simulink model "dual_mass_plant"  (R2023a)
settings: Solver=VariableStepAuto  StartTime=0.0  StopTime=50  RelTol=1e-3
values from neighbouring files (symbols this model uses):
  C = [1 0 1 0]    [dual_param.m]
  Kf1 = 2.0    (= 2)    [dual_param.m]
  Kf2 = 10.0    (= 10)    [dual_param.m]
  Kv1 = 0.1    [dual_param.m]
  Kv2 = 0.5    [dual_param.m]
  M = 10.0    (= 10)    [dual_param.m]
  m = 1.0    (= 1)    [dual_param.m]
  U1 = 1.0    (= 1)    [dual_param.m]
  U2 = 3.0    (= 3)    [dual_param.m]
settings Model: Creator=Admin  LastModifiedBy=Admin
settings ModelReferenceCC: EnableRefExpFcnMdlSchedulingChecks=on

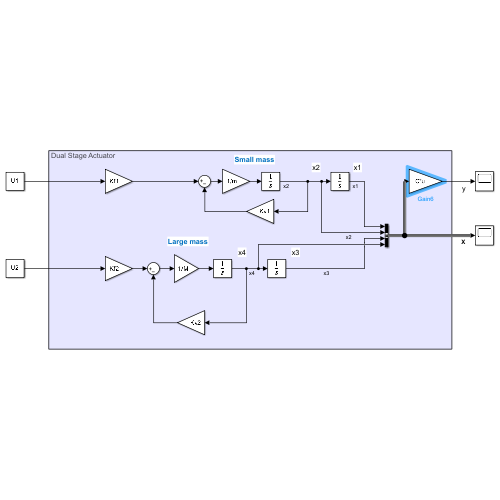
[thumbnail: Simulink's stored preview of the top-level diagram]
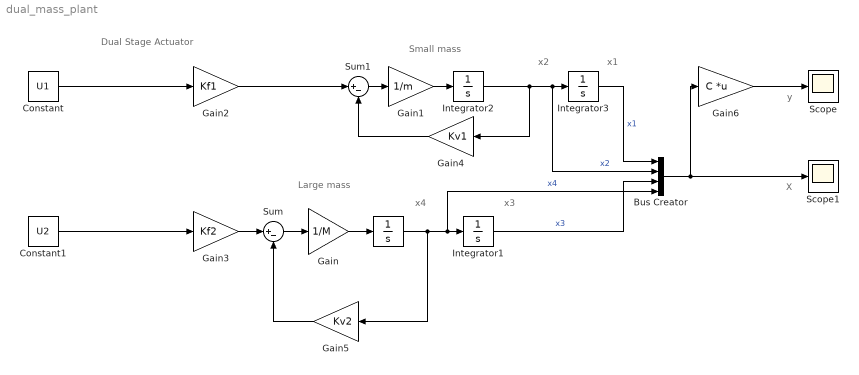
== system dual_mass_plant ==
  note: X
  note: Dual Stage Actuator
  note: y
  note: Small mass
  note: Large mass
  note: x1
  note: x2
  note: x3
  note: x4
  " " : Integrator
  Bus Creator : BusCreator  Inputs=4
  Constant : Constant  Value=U1
  Constant1 : Constant  Value=U2
  Gain : Gain  Gain=1/M
  Gain1 : Gain  Gain=1/m
  Gain2 : Gain  Gain=Kf1
  Gain3 : Gain  Gain=Kf2
  Gain4 : Gain  Gain=Kv1
  Gain5 : Gain  Gain=Kv2
  Gain6 : Gain  Gain=C  Multiplication=Matrix(K*u)
  Integrator1 : Integrator
  Integrator2 : Integrator
  Integrator3 : Integrator
  Scope : Scope
  Scope1 : Scope
  Sum : Sum  Inputs=|+-
  Sum1 : Sum  Inputs=|+-
  wires:
  Integrator2/1 -> Bus Creator/2, Integrator3/1, Gain4/1  "x2"
  " "/1 -> Gain5/1, Bus Creator/4, Integrator1/1  "x4"
  Gain/1 -> " "/1
  Sum/1 -> Gain/1
  Integrator3/1 -> Bus Creator/1  "x1"
  Integrator1/1 -> Bus Creator/3  "x3"
  Gain3/1 -> Sum/1
  Sum1/1 -> Gain1/1
  Gain1/1 -> Integrator2/1
  Gain4/1 -> Sum1/2
  Gain5/1 -> Sum/2
  Gain2/1 -> Sum1/1
  Bus Creator/1 -> Gain6/1, Scope1/1
  Constant/1 -> Gain2/1
  Constant1/1 -> Gain3/1
  Gain6/1 -> Scope/1
